simulink model "HighClearancePlant"  (R2016b)
settings: Solver=FixedStepAuto  StartTime=0.0  StopTime=runTime  FixedStep=step_time  MaxStep=0.05  RelTol=1e-3
PreLoadFcn:
  | %load('PlantConfig.mat');
  | run 'PlantParams.m';
values from neighbouring files (symbols this model uses):
  coilMaxI = 0.9*amp2mAmp*Vs/coilR    (= 1800)    [PlantParams.m]
  coilMinI = 0.2*amp2mAmp*Vs/coilR    (= 400)    [PlantParams.m]
  maxFlowRate = maxFlowRate*1    (= 16)    [PlantParams.m]
  reducer_ex = 0.01    [PlantParams.m]
  reducer_rt = 0.01    [PlantParams.m]
  strokeLegnth = 500    [PlantParams.m]
  Vs = 12    [PlantParams.m]
undefined symbols (not defined in the file or in its folder): DiscIntNeverNeededParam, IOD_OK, positionSensor_tblData, positionSensorFL_BrkPnts, positionSensorFR_BrkPnts, positionSensorRL_BrkPnts, positionSensorRR_BrkPnts, trackWidthMin, twoWheelSteer
undefined symbols (not defined in the file): dampeningFL, dampeningFR, extendRateFL, extendRateFR, retractRateFL, retractRateFR
libraries: HighClearance_library x14, PlantLibrary x14, simulink x4
settings Model: Creator=lemaya  LastModifiedBy=lemaya
settings OptimizationCC: DefaultUnderspecifiedDataType=single
settings DebuggingCC: FrameProcessingCompatibilityMsg=warning

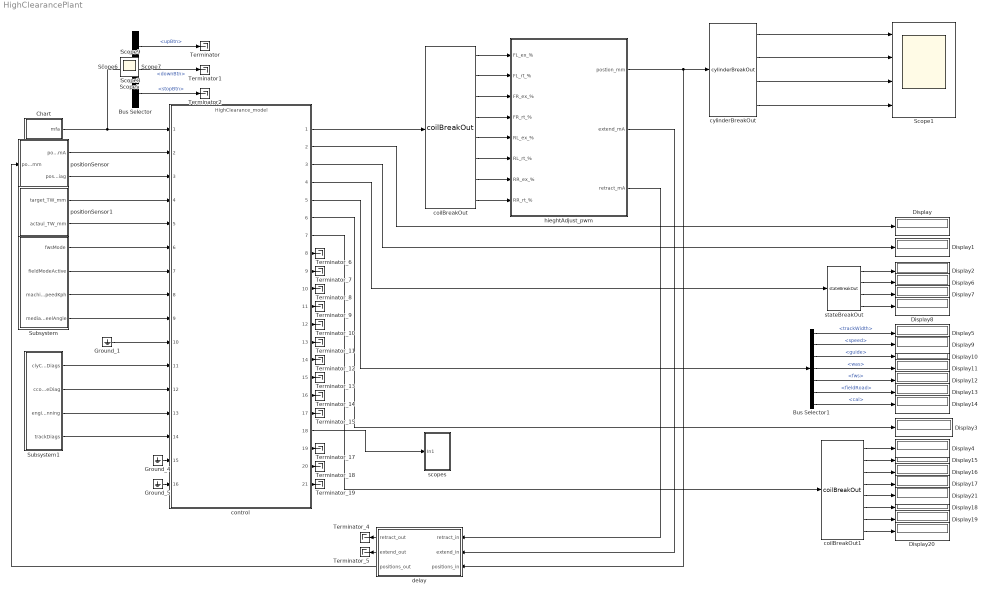
== system HighClearancePlant ==
  Bus Selector : BusSelector  OutputSignals=upBtn,downBtn,stopBtn
  Bus Selector1 : BusSelector  OutputSignals=trackWidth,speed,guide,was,fws,fieldRoad,cal
  Chart : Stateflow chart  TreatAsAtomicUnit=on
  Display{,1..21} (22 alike) : Display
      Display3 settings: Format=hex (Stored Integer)
  Ground_1 : Ground
  Ground_4 : Ground
  Ground_5 : Ground
  Scope1 : Scope  NumInputPorts=4
  Subsystem : Subsystem
  Subsystem1 : Subsystem
  Terminator : Terminator
  Terminator1 : Terminator
  Terminator2 : Terminator
  Terminator_{4..15,17..19} (15 alike) : Terminator
  coilBreakOut : HighClearance_library/coilBreakOut
  coilBreakOut1 : HighClearance_library/coilBreakOut
  control : ModelReference  ModelNameDialog=HighClearance_model.slx  SimulationMode=Normal  ModelReferenceVersion=1.415
  cylinderBreakOut : HighClearance_library/cylinderBreakOut
  delay : Subsystem
  hieghtAdjust_pwm : Subsystem  AncestorBlock=PlantLibrary/hieghtAdjust_pwm
  positionSensor : Subsystem
  positionSensor1 : Subsystem
  scopes : Subsystem
  stateBreakOut : HighClearance_library/stateBreakOut
  Scope{,2..9} (9 alike) : Scope
  wires:
  hieghtAdjust_pwm/2(extend_mA) -> delay/2(extend_in)
  hieghtAdjust_pwm/3(retract_mA) -> delay/1(retract_in)
  hieghtAdjust_pwm/1(postion_mm) -> delay/3(positions_in), cylinderBreakOut/1
  control/1 -> coilBreakOut/1
  positionSensor/1(positions_mA) -> control/2
  delay/3(positions_out) -> positionSensor/1(positons_mm)
  Chart/1(mfa) -> Bus Selector/1, control/1
  coilBreakOut/2 -> hieghtAdjust_pwm/2(FL_rt_%)
  coilBreakOut/3 -> hieghtAdjust_pwm/3(FR_ex_%)
  coilBreakOut/4 -> hieghtAdjust_pwm/4(FR_rt_%)
  coilBreakOut/5 -> hieghtAdjust_pwm/5(RL_ex_%)
  coilBreakOut/6 -> hieghtAdjust_pwm/6(RL_rt_%)
  coilBreakOut/7 -> hieghtAdjust_pwm/7(RR_ex_%)
  coilBreakOut/8 -> hieghtAdjust_pwm/8(RR_rt_%)
  coilBreakOut/1 -> hieghtAdjust_pwm/1(FL_ex_%)
  positionSensor/2(positions_diag) -> control/3
  positionSensor1/1(target_TW_mm) -> control/4
  positionSensor1/2(actaul_TW_mm) -> control/5
  Subsystem/1(fwsMode) -> control/6
  Subsystem/2(fieldModeActive) -> control/7
  Subsystem/3(machineSpeedKph) -> control/8
  Subsystem/4(medianWheelAngle) -> control/9
  Subsystem1/1(clyCoilDiags) -> control/11
  Subsystem1/2(ccoEnableDiag) -> control/12
  control/2 -> Display/1
  control/3 -> Display1/1
  control/4 -> stateBreakOut/1
  control/6 -> Display3/1
  control/7 -> coilBreakOut1/1
  control/5 -> Bus Selector1/1
  Bus Selector/1 -> Terminator/1  "<upBtn>"
  Bus Selector/2 -> Terminator1/1  "<downBtn>"
  Bus Selector/3 -> Terminator2/1  "<stopBtn>"
  Ground_1/1 -> control/10
  delay/1(retract_out) -> Terminator_4/1
  delay/2(extend_out) -> Terminator_5/1
  stateBreakOut/1 -> Display2/1
  stateBreakOut/2 -> Display6/1
  stateBreakOut/3 -> Display7/1
  stateBreakOut/4 -> Display8/1
  Bus Selector1/1 -> Display5/1  "<trackWidth>"
  Bus Selector1/2 -> Display9/1  "<speed>"
  Bus Selector1/3 -> Display10/1  "<guide>"
  Bus Selector1/4 -> Display11/1  "<was>"
  Bus Selector1/5 -> Display12/1  "<fws>"
  Bus Selector1/6 -> Display13/1  "<fieldRoad>"
  Bus Selector1/7 -> Display14/1  "<cal>"
  coilBreakOut1/1 -> Display4/1
  coilBreakOut1/2 -> Display15/1
  coilBreakOut1/3 -> Display16/1
  coilBreakOut1/4 -> Display17/1
  coilBreakOut1/8 -> Display20/1
  coilBreakOut1/7 -> Display19/1
  coilBreakOut1/6 -> Display18/1
  coilBreakOut1/5 -> Display21/1
  cylinderBreakOut/3 -> Scope1/3
  cylinderBreakOut/4 -> Scope1/4
  cylinderBreakOut/2 -> Scope1/2
  cylinderBreakOut/1 -> Scope1/1
  Ground_4/1 -> control/15
  Ground_5/1 -> control/16
  control/8 -> Terminator_6/1
  control/9 -> Terminator_7/1
  control/10 -> Terminator_8/1
  control/11 -> Terminator_9/1
  control/12 -> Terminator_10/1
  control/13 -> Terminator_11/1
  control/14 -> Terminator_12/1
  control/15 -> Terminator_13/1
  control/16 -> Terminator_14/1
  control/17 -> Terminator_15/1
  control/19 -> Terminator_17/1
  control/20 -> Terminator_18/1
  control/21 -> Terminator_19/1
  Subsystem1/3(engineRunning) -> control/13
  Subsystem1/4(trackDiags) -> control/14
  control/18 -> scopes/1(In1)

== system HighClearancePlant/Subsystem ==
  Constant : Constant  Value=twoWheelSteer
  Constant1 : Constant  OutDataTypeStr=Inherit: Inherit via back propagation
  Constant2 : Constant  Value=5  OutDataTypeStr=Inherit: Inherit via back propagation
  Constant3 : Constant  Value=0  OutDataTypeStr=Inherit: Inherit via back propagation
  fwsMode : Outport
  fieldModeActive : Outport  Port=2
  machineSpeedKph : Outport  Port=3
  medianWheelAngle : Outport  Port=4
  wires:
  Constant/1 -> fwsMode/1
  Constant1/1 -> fieldModeActive/1
  Constant2/1 -> machineSpeedKph/1
  Constant3/1 -> medianWheelAngle/1

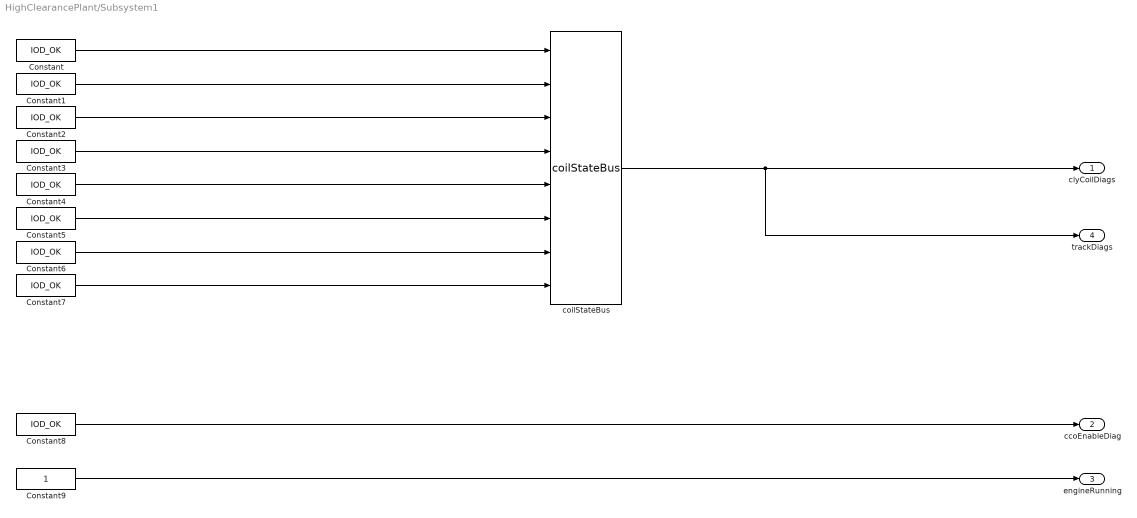
== system HighClearancePlant/Subsystem1 ==
  Constant{,1..8} (9 alike) : Constant  Value=IOD_OK
  Constant9 : Constant  OutDataTypeStr=boolean
  coilStateBus : HighClearance_library/coilStateBus
  clyCoilDiags : Outport
  ccoEnableDiag : Outport  Port=2
  engineRunning : Outport  Port=3
  trackDiags : Outport  Port=4
  wires:
  Constant/1 -> coilStateBus/1
  Constant1/1 -> coilStateBus/2
  Constant2/1 -> coilStateBus/3
  Constant3/1 -> coilStateBus/4
  Constant4/1 -> coilStateBus/5
  Constant5/1 -> coilStateBus/6
  Constant6/1 -> coilStateBus/7
  Constant7/1 -> coilStateBus/8
  coilStateBus/1 -> trackDiags/1, clyCoilDiags/1
  Constant8/1 -> ccoEnableDiag/1
  Constant9/1 -> engineRunning/1

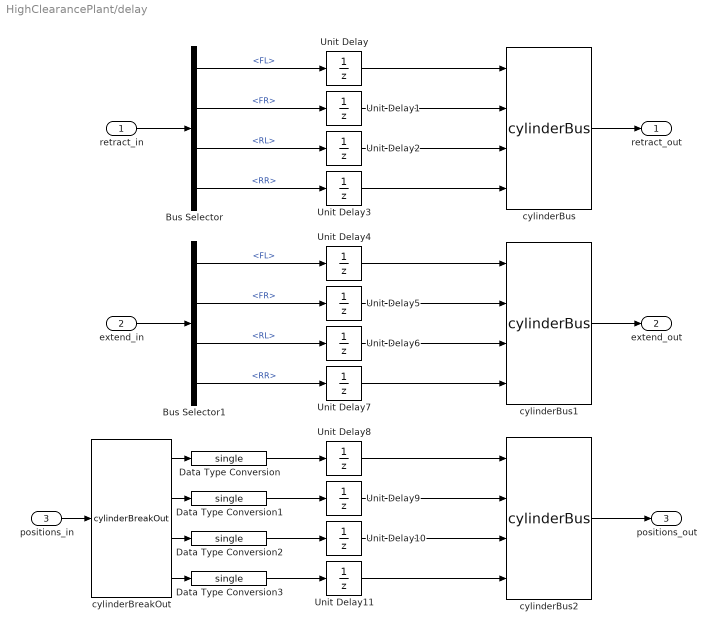
== system HighClearancePlant/delay ==
  retract_in : Inport
  extend_in : Inport  Port=2
  positions_in : Inport  Port=3
  Bus Selector : BusSelector  OutputSignals=FL,FR,RL,RR
  Bus Selector1 : BusSelector  OutputSignals=FL,FR,RL,RR
  Data Type Conversion{,1..3} (4 alike) : DataTypeConversion  OutDataTypeStr=single
  Unit Delay{,1..11} (12 alike) : UnitDelay  SampleTime=-1
  cylinderBreakOut : HighClearance_library/cylinderBreakOut
  cylinderBus : HighClearance_library/cylinderBus
  cylinderBus1 : HighClearance_library/cylinderBus
  cylinderBus2 : HighClearance_library/cylinderBus
  retract_out : Outport
  extend_out : Outport  Port=2
  positions_out : Outport  Port=3
  wires:
  cylinderBus/1 -> retract_out/1
  cylinderBus1/1 -> extend_out/1
  cylinderBus2/1 -> positions_out/1
  retract_in/1 -> Bus Selector/1
  extend_in/1 -> Bus Selector1/1
  Bus Selector1/4 -> Unit Delay7/1  "<RR>"
  Bus Selector1/2 -> Unit Delay5/1  "<FR>"
  Bus Selector1/1 -> Unit Delay4/1  "<FL>"
  Bus Selector1/3 -> Unit Delay6/1  "<RL>"
  Bus Selector/4 -> Unit Delay3/1  "<RR>"
  Bus Selector/1 -> Unit Delay/1  "<FL>"
  Bus Selector/3 -> Unit Delay2/1  "<RL>"
  Bus Selector/2 -> Unit Delay1/1  "<FR>"
  Unit Delay/1 -> cylinderBus/1
  Unit Delay1/1 -> cylinderBus/2
  Unit Delay2/1 -> cylinderBus/3
  Unit Delay3/1 -> cylinderBus/4
  Unit Delay4/1 -> cylinderBus1/1
  Unit Delay7/1 -> cylinderBus1/4
  Unit Delay6/1 -> cylinderBus1/3
  Unit Delay5/1 -> cylinderBus1/2
  Unit Delay8/1 -> cylinderBus2/1
  Unit Delay9/1 -> cylinderBus2/2
  Unit Delay10/1 -> cylinderBus2/3
  Unit Delay11/1 -> cylinderBus2/4
  Data Type Conversion/1 -> Unit Delay8/1
  Data Type Conversion1/1 -> Unit Delay9/1
  Data Type Conversion2/1 -> Unit Delay10/1
  Data Type Conversion3/1 -> Unit Delay11/1
  positions_in/1 -> cylinderBreakOut/1
  cylinderBreakOut/1 -> Data Type Conversion/1
  cylinderBreakOut/2 -> Data Type Conversion1/1
  cylinderBreakOut/3 -> Data Type Conversion2/1
  cylinderBreakOut/4 -> Data Type Conversion3/1

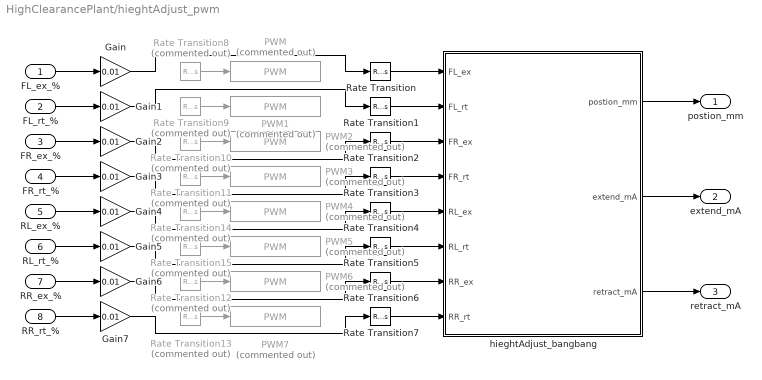
== system HighClearancePlant/hieghtAdjust_pwm ==
  FL_ex_% : Inport
  FL_rt_% : Inport  Port=2
  FR_ex_% : Inport  Port=3
  FR_rt_% : Inport  Port=4
  RL_ex_% : Inport  Port=5
  RL_rt_% : Inport  Port=6
  RR_ex_% : Inport  Port=7
  RR_rt_% : Inport  Port=8
  Gain{,1..7} (8 alike) : Gain  Gain=0.01
  PWM{,1..7} (8 alike) : PlantLibrary/PWM  Commented=on
  Rate Transition{,1..7} (8 alike) : RateTransition
  Rate Transition{8..15} (8 alike) : RateTransition  Commented=on  OutPortSampleTime=0.0001
  hieghtAdjust_bangbang : Subsystem  AncestorBlock=PlantLibrary/hieghtAdjust_bangbang
  postion_mm : Outport
  extend_mA : Outport  Port=2
  retract_mA : Outport  Port=3
  wires:
  Rate Transition7/1 -> hieghtAdjust_bangbang/8(RR_rt)
  Rate Transition6/1 -> hieghtAdjust_bangbang/7(RR_ex)
  Rate Transition5/1 -> hieghtAdjust_bangbang/6(RL_rt)
  Rate Transition4/1 -> hieghtAdjust_bangbang/5(RL_ex)
  Rate Transition3/1 -> hieghtAdjust_bangbang/4(FR_rt)
  Rate Transition2/1 -> hieghtAdjust_bangbang/3(FR_ex)
  Rate Transition1/1 -> hieghtAdjust_bangbang/2(FL_rt)
  Rate Transition/1 -> hieghtAdjust_bangbang/1(FL_ex)
  hieghtAdjust_bangbang/2(extend_mA) -> extend_mA/1
  hieghtAdjust_bangbang/3(retract_mA) -> retract_mA/1
  hieghtAdjust_bangbang/1(postion_mm) -> postion_mm/1
  Rate Transition8/1 -> PWM/1
  Rate Transition9/1 -> PWM1/1
  Rate Transition10/1 -> PWM2/1
  Rate Transition11/1 -> PWM3/1
  Rate Transition14/1 -> PWM4/1
  Rate Transition15/1 -> PWM5/1
  Rate Transition12/1 -> PWM6/1
  Rate Transition13/1 -> PWM7/1
  FL_ex_%/1 -> Gain/1
  FL_rt_%/1 -> Gain1/1
  Gain1/1 -> Rate Transition1/1
  Gain/1 -> Rate Transition/1
  FR_ex_%/1 -> Gain2/1
  Gain2/1 -> Rate Transition2/1
  FR_rt_%/1 -> Gain3/1
  Gain3/1 -> Rate Transition3/1
  RL_ex_%/1 -> Gain4/1
  Gain4/1 -> Rate Transition4/1
  RL_rt_%/1 -> Gain5/1
  Gain5/1 -> Rate Transition5/1
  RR_ex_%/1 -> Gain6/1
  Gain6/1 -> Rate Transition6/1
  RR_rt_%/1 -> Gain7/1
  Gain7/1 -> Rate Transition7/1

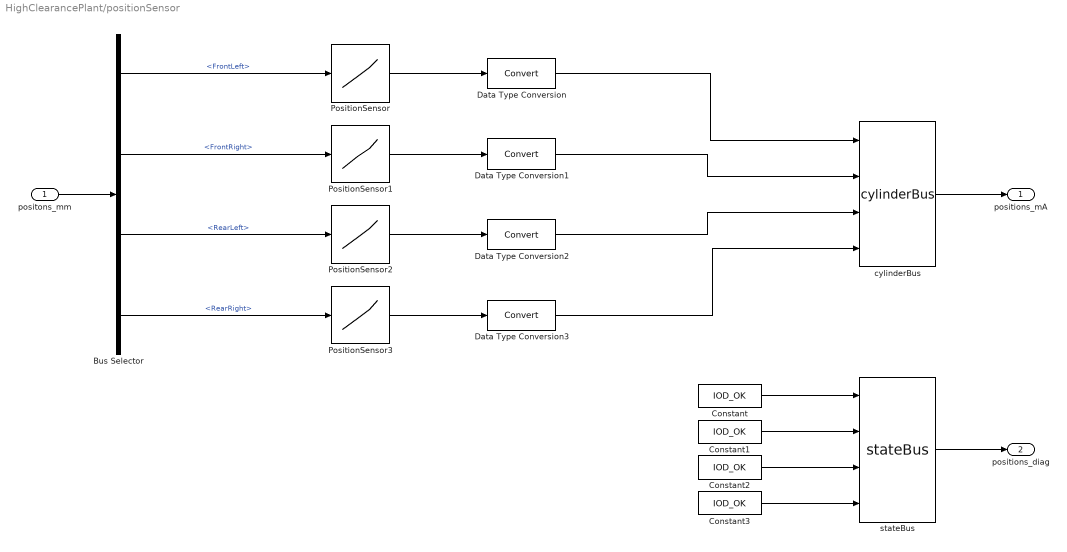
== system HighClearancePlant/positionSensor ==
  positons_mm : Inport
  Bus Selector : BusSelector  OutputSignals=FrontLeft,FrontRight,RearLeft,RearRight
  Constant{,1..3} (4 alike) : Constant  Value=IOD_OK
  Data Type Conversion{,1..3} (4 alike) : DataTypeConversion
  PositionSensor : Lookup_n-D  NumberOfTableDimensions=1  BreakpointsForDimension1=positionSensor_tblData  Table=positionSensorFL_BrkPnts  ExtrapMethod=Clip  UseLastTableValue=on  InternalRulePriority=Speed  RndMeth=Simplest  InputSameDT=on
  PositionSensor1 : Lookup_n-D  NumberOfTableDimensions=1  BreakpointsForDimension1=positionSensor_tblData  Table=positionSensorFR_BrkPnts  ExtrapMethod=Clip  UseLastTableValue=on  InternalRulePriority=Speed  RndMeth=Simplest  InputSameDT=on
  PositionSensor2 : Lookup_n-D  NumberOfTableDimensions=1  BreakpointsForDimension1=positionSensor_tblData  Table=positionSensorRL_BrkPnts  ExtrapMethod=Clip  UseLastTableValue=on  InternalRulePriority=Speed  RndMeth=Simplest  InputSameDT=on
  PositionSensor3 : Lookup_n-D  NumberOfTableDimensions=1  BreakpointsForDimension1=positionSensor_tblData  Table=positionSensorRR_BrkPnts  ExtrapMethod=Clip  UseLastTableValue=on  InternalRulePriority=Speed  RndMeth=Simplest  InputSameDT=on
  cylinderBus : HighClearance_library/cylinderBus
  stateBus : HighClearance_library/stateBus
  positions_mA : Outport  OutDataTypeStr=Bus: CylinderBus
  positions_diag : Outport  Port=2  OutDataTypeStr=Bus: StateBus
  wires:
  positons_mm/1 -> Bus Selector/1
  Bus Selector/1 -> PositionSensor/1  "<FrontLeft>"
  Bus Selector/2 -> PositionSensor1/1  "<FrontRight>"
  Bus Selector/3 -> PositionSensor2/1  "<RearLeft>"
  Bus Selector/4 -> PositionSensor3/1  "<RearRight>"
  PositionSensor/1 -> Data Type Conversion/1
  PositionSensor1/1 -> Data Type Conversion1/1
  PositionSensor2/1 -> Data Type Conversion2/1
  PositionSensor3/1 -> Data Type Conversion3/1
  Data Type Conversion/1 -> cylinderBus/1
  Data Type Conversion1/1 -> cylinderBus/2
  Data Type Conversion2/1 -> cylinderBus/3
  Data Type Conversion3/1 -> cylinderBus/4
  cylinderBus/1 -> positions_mA/1
  stateBus/1 -> positions_diag/1
  Constant/1 -> stateBus/1
  Constant1/1 -> stateBus/2
  Constant2/1 -> stateBus/3
  Constant3/1 -> stateBus/4

== system HighClearancePlant/positionSensor1 ==
  Constant : Constant  Value=trackWidthMin  OutDataTypeStr=Inherit: Inherit via back propagation
  cylinderBus : HighClearance_library/cylinderBus
  cylinderBus1 : HighClearance_library/cylinderBus
  target_TW_mm : Outport  OutDataTypeStr=Bus: CylinderBus
  actaul_TW_mm : Outport  Port=2  OutDataTypeStr=Bus: CylinderBus
  wires:
  cylinderBus1/1 -> actaul_TW_mm/1
  cylinderBus/1 -> target_TW_mm/1
  Constant/1 -> cylinderBus1/4, cylinderBus1/3, cylinderBus1/2, cylinderBus1/1, cylinderBus/4, cylinderBus/3, cylinderBus/2, cylinderBus/1

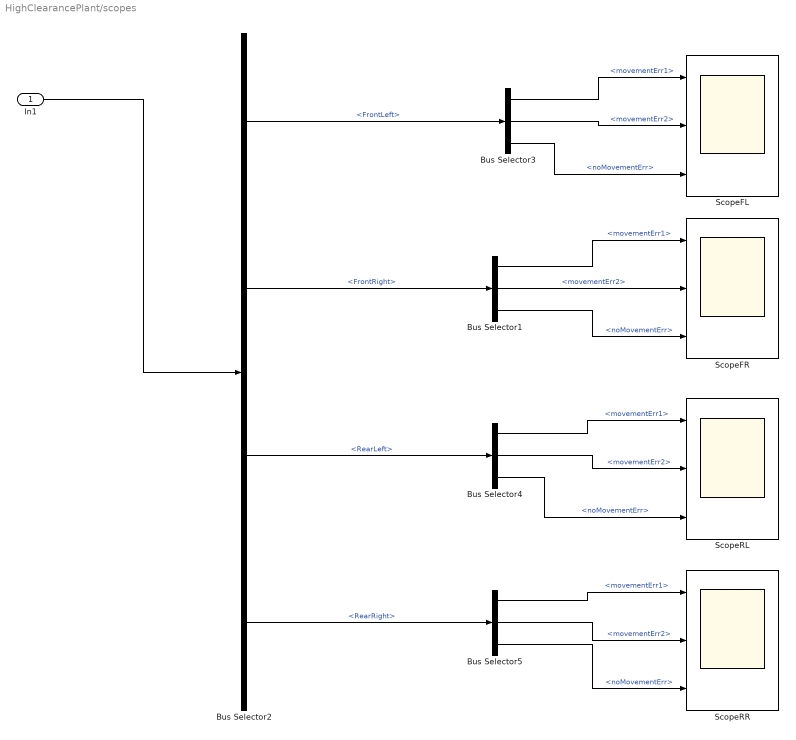
== system HighClearancePlant/scopes ==
  In1 : Inport
  Bus Selector{1,3..5} (4 alike) : BusSelector  OutputSignals=movementErr1,movementErr2,noMovementErr
  Bus Selector2 : BusSelector  OutputSignals=FrontLeft,FrontRight,RearLeft,RearRight
  ScopeFL : Scope  NumInputPorts=3
  ScopeFR : Scope  NumInputPorts=3
  ScopeRL : Scope  NumInputPorts=3
  ScopeRR : Scope  NumInputPorts=3
  wires:
  In1/1 -> Bus Selector2/1
  Bus Selector2/1 -> Bus Selector3/1  "<FrontLeft>"
  Bus Selector2/2 -> Bus Selector1/1  "<FrontRight>"
  Bus Selector2/3 -> Bus Selector4/1  "<RearLeft>"
  Bus Selector2/4 -> Bus Selector5/1  "<RearRight>"
  Bus Selector3/2 -> ScopeFL/2  "<movementErr2>"
  Bus Selector3/1 -> ScopeFL/1  "<movementErr1>"
  Bus Selector3/3 -> ScopeFL/3  "<noMovementErr>"
  Bus Selector1/2 -> ScopeFR/2  "<movementErr2>"
  Bus Selector1/3 -> ScopeFR/3  "<noMovementErr>"
  Bus Selector1/1 -> ScopeFR/1  "<movementErr1>"
  Bus Selector4/2 -> ScopeRL/2  "<movementErr2>"
  Bus Selector4/1 -> ScopeRL/1  "<movementErr1>"
  Bus Selector4/3 -> ScopeRL/3  "<noMovementErr>"
  Bus Selector5/1 -> ScopeRR/1  "<movementErr1>"
  Bus Selector5/2 -> ScopeRR/2  "<movementErr2>"
  Bus Selector5/3 -> ScopeRR/3  "<noMovementErr>"

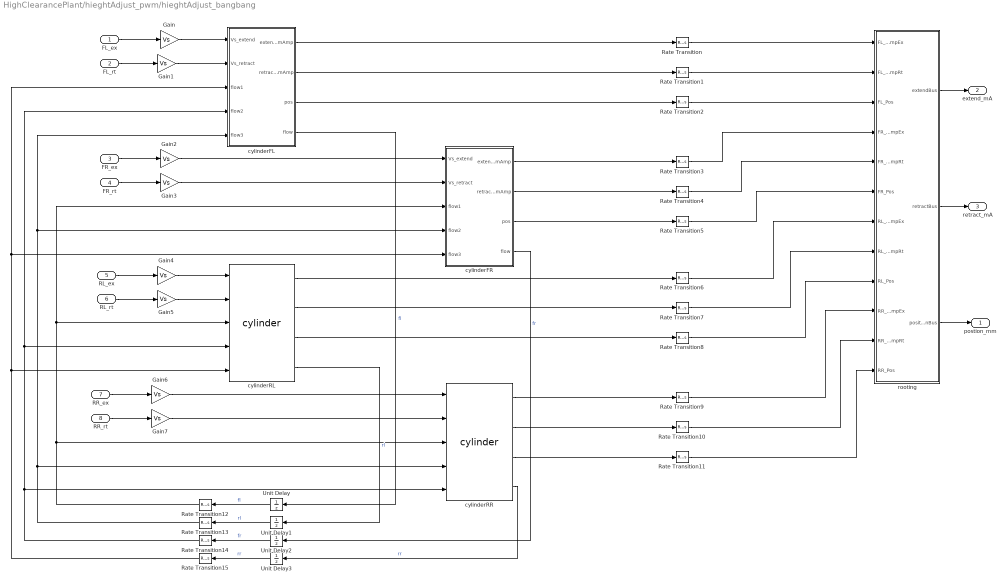
== system HighClearancePlant/hieghtAdjust_pwm/hieghtAdjust_bangbang ==
  FL_ex : Inport
  FL_rt : Inport  Port=2
  FR_ex : Inport  Port=3
  FR_rt : Inport  Port=4
  RL_ex : Inport  Port=5
  RL_rt : Inport  Port=6
  RR_ex : Inport  Port=7
  RR_rt : Inport  Port=8
  Gain{,1..7} (8 alike) : Gain  Gain=Vs
  Rate Transition{,1..11,13..15} (15 alike) : RateTransition  OutPortSampleTime=step_time
  Rate Transition12 : RateTransition
  Unit Delay{,1..3} (4 alike) : UnitDelay  SampleTime=-1
  cylinderFL : Subsystem  AncestorBlock=PlantLibrary/cylinder  mask{dampening=dampeningFL, extendRate=extendRateFL, retractRate=retractRateFL}
      mask prompts: dampening "Dampening coefficient:"; extendRate "Extend Rate [mm/sec]:"; retractRate "Retract Rate [mm/sec]:"
  cylinderFR : Subsystem  AncestorBlock=PlantLibrary/cylinder  mask{dampening=dampeningFR, extendRate=extendRateFR, retractRate=retractRateFR}
      mask prompts: dampening "Dampening coefficient:"; extendRate "Extend Rate [mm/sec]:"; retractRate "Retract Rate [mm/sec]:"
  cylinderRL : PlantLibrary/cylinder  dampening=dampeningRL  extendRate=extendRateRL  retractRate=retractRateRL
  cylinderRR : PlantLibrary/cylinder  dampening=dampeningRR  extendRate=extendRateRR  retractRate=retractRateRR
  rooting : Subsystem
  postion_mm : Outport
  extend_mA : Outport  Port=2
  retract_mA : Outport  Port=3
  wires:
  cylinderRR/2 -> Rate Transition10/1
  cylinderRR/1 -> Rate Transition9/1
  cylinderRL/2 -> Rate Transition7/1
  cylinderRL/1 -> Rate Transition6/1
  cylinderFR/2(retract_mAmp) -> Rate Transition4/1
  cylinderFR/1(extend_mAmp) -> Rate Transition3/1
  cylinderFL/2(retract_mAmp) -> Rate Transition1/1
  cylinderFL/1(extend_mAmp) -> Rate Transition/1
  rooting/3(positionBus) -> postion_mm/1
  rooting/2(retractBus) -> retract_mA/1
  rooting/1(extendBus) -> extend_mA/1
  FL_rt/1 -> Gain1/1
  RR_rt/1 -> Gain7/1
  RL_ex/1 -> Gain4/1
  FL_ex/1 -> Gain/1
  FR_ex/1 -> Gain2/1
  FR_rt/1 -> Gain3/1
  RR_ex/1 -> Gain6/1
  RL_rt/1 -> Gain5/1
  Gain/1 -> cylinderFL/1(Vs_extend)
  Gain1/1 -> cylinderFL/2(Vs_retract)
  Gain4/1 -> cylinderRL/1
  Gain5/1 -> cylinderRL/2
  Gain6/1 -> cylinderRR/1
  Gain7/1 -> cylinderRR/2
  Rate Transition/1 -> rooting/1(FL_mAmpEx)
  Rate Transition1/1 -> rooting/2(FL_mAmpRt)
  Rate Transition2/1 -> rooting/3(FL_Pos)
  Rate Transition3/1 -> rooting/4(FR_mAmpEx)
  Rate Transition4/1 -> rooting/5(FR_mAmpRt)
  Rate Transition5/1 -> rooting/6(FR_Pos)
  Rate Transition6/1 -> rooting/7(RL_mAmpEx)
  Rate Transition7/1 -> rooting/8(RL_mAmpRt)
  Rate Transition8/1 -> rooting/9(RL_Pos)
  Rate Transition9/1 -> rooting/10(RR_mAmpEx)
  Rate Transition10/1 -> rooting/11(RR_mAmpRt)
  Rate Transition11/1 -> rooting/12(RR_Pos)
  cylinderFL/3(pos) -> Rate Transition2/1
  cylinderRL/3 -> Rate Transition8/1
  cylinderFR/3(pos) -> Rate Transition5/1
  cylinderRR/3 -> Rate Transition11/1
  Gain3/1 -> cylinderFR/2(Vs_retract)
  Gain2/1 -> cylinderFR/1(Vs_extend)
  cylinderRL/4 -> Unit Delay1/1  "rl"
  cylinderFR/4(flow) -> Unit Delay2/1  "fr"
  cylinderRR/4 -> Unit Delay3/1  "rr"
  cylinderFL/4(flow) -> Unit Delay/1  "fl"
  Unit Delay/1 -> Rate Transition12/1  "fl"
  Unit Delay3/1 -> Rate Transition15/1  "rr"
  Unit Delay2/1 -> Rate Transition14/1  "fr"
  Unit Delay1/1 -> Rate Transition13/1  "rl"
  Rate Transition12/1 -> cylinderFR/3(flow1), cylinderRL/3, cylinderRR/3
  Rate Transition13/1 -> cylinderFL/5(flow3), cylinderFR/4(flow2), cylinderRR/4
  Rate Transition14/1 -> cylinderFL/4(flow2), cylinderRL/4, cylinderRR/5
  Rate Transition15/1 -> cylinderRL/5, cylinderFL/3(flow1), cylinderFR/5(flow3)

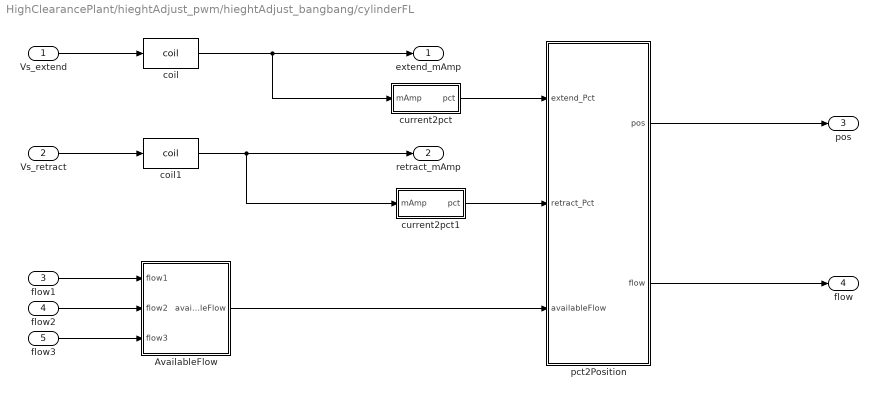
== system HighClearancePlant/hieghtAdjust_pwm/hieghtAdjust_bangbang/cylinderFL ==
  Vs_extend : Inport
  Vs_retract : Inport  Port=2
  flow1 : Inport  Port=3
  flow2 : Inport  Port=4
  flow3 : Inport  Port=5
  AvailableFlow : Subsystem
  coil : PlantLibrary/coil
  coil1 : PlantLibrary/coil
  current2pct : Subsystem
  current2pct1 : Subsystem
  pct2Position : Subsystem
  extend_mAmp : Outport
  retract_mAmp : Outport  Port=2
  pos : Outport  Port=3
  flow : Outport  Port=4
  wires:
  Vs_extend/1 -> coil/1
  Vs_retract/1 -> coil1/1
  coil/1 -> current2pct/1(mAmp), extend_mAmp/1
  coil1/1 -> current2pct1/1(mAmp), retract_mAmp/1
  current2pct/1(pct) -> pct2Position/1(extend_Pct)
  current2pct1/1(pct) -> pct2Position/2(retract_Pct)
  pct2Position/1(pos) -> pos/1
  pct2Position/2(flow) -> flow/1
  flow1/1 -> AvailableFlow/1(flow1)
  flow2/1 -> AvailableFlow/2(flow2)
  flow3/1 -> AvailableFlow/3(flow3)
  AvailableFlow/1(availableFlow) -> pct2Position/3(availableFlow)

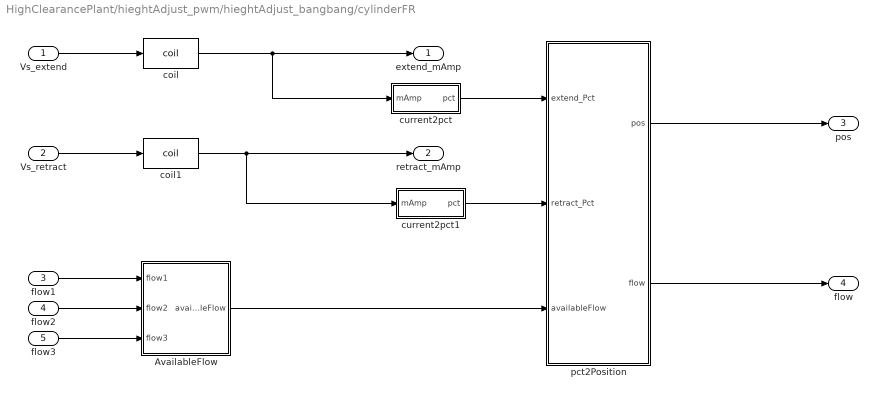
== system HighClearancePlant/hieghtAdjust_pwm/hieghtAdjust_bangbang/cylinderFR ==
  Vs_extend : Inport
  Vs_retract : Inport  Port=2
  flow1 : Inport  Port=3
  flow2 : Inport  Port=4
  flow3 : Inport  Port=5
  AvailableFlow : Subsystem
  coil : PlantLibrary/coil
  coil1 : PlantLibrary/coil
  current2pct : Subsystem
  current2pct1 : Subsystem
  pct2Position : Subsystem
  extend_mAmp : Outport
  retract_mAmp : Outport  Port=2
  pos : Outport  Port=3
  flow : Outport  Port=4
  wires:
  Vs_extend/1 -> coil/1
  Vs_retract/1 -> coil1/1
  coil/1 -> current2pct/1(mAmp), extend_mAmp/1
  coil1/1 -> current2pct1/1(mAmp), retract_mAmp/1
  current2pct/1(pct) -> pct2Position/1(extend_Pct)
  current2pct1/1(pct) -> pct2Position/2(retract_Pct)
  pct2Position/1(pos) -> pos/1
  pct2Position/2(flow) -> flow/1
  flow1/1 -> AvailableFlow/1(flow1)
  flow2/1 -> AvailableFlow/2(flow2)
  flow3/1 -> AvailableFlow/3(flow3)
  AvailableFlow/1(availableFlow) -> pct2Position/3(availableFlow)

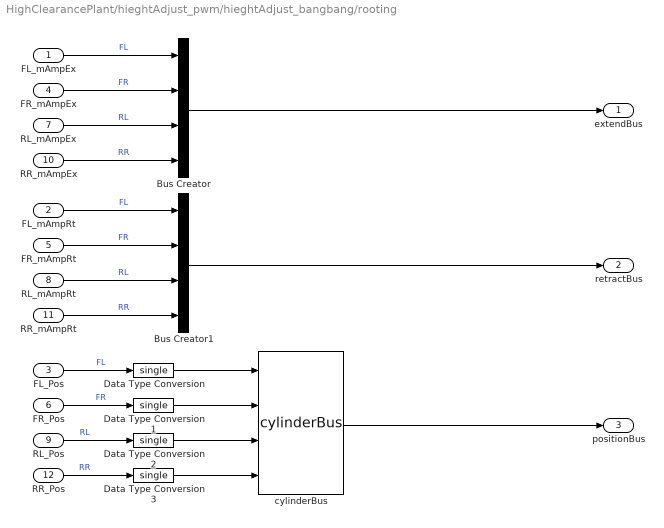
== system HighClearancePlant/hieghtAdjust_pwm/hieghtAdjust_bangbang/rooting ==
  FL_mAmpEx : Inport
  FL_mAmpRt : Inport  Port=2
  FL_Pos : Inport  Port=3
  FR_mAmpEx : Inport  Port=4
  FR_mAmpRt : Inport  Port=5
  FR_Pos : Inport  Port=6
  RL_mAmpEx : Inport  Port=7
  RL_mAmpRt : Inport  Port=8
  RL_Pos : Inport  Port=9
  RR_mAmpEx : Inport  Port=10
  RR_mAmpRt : Inport  Port=11
  RR_Pos : Inport  Port=12
  Bus Creator : BusCreator  Inputs=4
  Bus Creator1 : BusCreator  Inputs=4
  Data Type Conversion{,1..3} (4 alike) : DataTypeConversion  OutDataTypeStr=single
  cylinderBus : HighClearance_library/cylinderBus
  extendBus : Outport
  retractBus : Outport  Port=2
  positionBus : Outport  Port=3
  wires:
  Bus Creator1/1 -> retractBus/1
  Bus Creator/1 -> extendBus/1
  RR_mAmpRt/1 -> Bus Creator1/4  "RR"
  RL_mAmpRt/1 -> Bus Creator1/3  "RL"
  FR_mAmpRt/1 -> Bus Creator1/2  "FR"
  FL_mAmpRt/1 -> Bus Creator1/1  "FL"
  RR_mAmpEx/1 -> Bus Creator/4  "RR"
  RL_mAmpEx/1 -> Bus Creator/3  "RL"
  FR_mAmpEx/1 -> Bus Creator/2  "FR"
  FL_mAmpEx/1 -> Bus Creator/1  "FL"
  cylinderBus/1 -> positionBus/1
  Data Type Conversion/1 -> cylinderBus/1
  Data Type Conversion1/1 -> cylinderBus/2
  Data Type Conversion2/1 -> cylinderBus/3
  Data Type Conversion3/1 -> cylinderBus/4
  FL_Pos/1 -> Data Type Conversion/1  "FL"
  FR_Pos/1 -> Data Type Conversion1/1  "FR"
  RL_Pos/1 -> Data Type Conversion2/1  "RL"
  RR_Pos/1 -> Data Type Conversion3/1  "RR"

== system HighClearancePlant/hieghtAdjust_pwm/hieghtAdjust_bangbang/cylinderFL/AvailableFlow ==
  flow1 : Inport
  flow2 : Inport  Port=2
  flow3 : Inport  Port=3
  Constant : Constant  Value=maxFlowRate
  Saturation : Saturate  UpperLimit=0  LowerLimit=-inf
  Subtract : Sum  Inputs=+-
  Sum : Sum  Inputs=+++
  availableFlow : Outport
  wires:
  flow3/1 -> Sum/3
  flow1/1 -> Sum/1
  Constant/1 -> Subtract/1
  flow2/1 -> Sum/2
  Sum/1 -> Subtract/2
  Subtract/1 -> Saturation/1
  Saturation/1 -> availableFlow/1

== system HighClearancePlant/hieghtAdjust_pwm/hieghtAdjust_bangbang/cylinderFL/current2pct ==
  mAmp : Inport
  Divide1 : Product  Inputs=*/
  Gain : Gain  Gain=100
  Relational Operator : RelationalOperator  OutDataTypeStr=boolean  RndMeth=Simplest
  Saturation : Saturate  UpperLimit=100  LowerLimit=0
  Switch : Switch  Criteria=u2 > Threshold
  maxCurrent : Constant  Value=coilMaxI
  minCurrent : Constant  Value=coilMinI
  pct : Outport
  wires:
  maxCurrent/1 -> Divide1/2
  Relational Operator/1 -> Switch/3, Switch/2
  minCurrent/1 -> Relational Operator/2
  Switch/1 -> Divide1/1
  mAmp/1 -> Relational Operator/1, Switch/1
  Divide1/1 -> Gain/1
  Saturation/1 -> pct/1
  Gain/1 -> Saturation/1

== system HighClearancePlant/hieghtAdjust_pwm/hieghtAdjust_bangbang/cylinderFL/current2pct1 ==
  mAmp : Inport
  Divide1 : Product  Inputs=*/
  Gain : Gain  Gain=100
  Relational Operator : RelationalOperator  OutDataTypeStr=boolean  RndMeth=Simplest
  Saturation : Saturate  UpperLimit=100  LowerLimit=0
  Switch : Switch  Criteria=u2 > Threshold
  maxCurrent : Constant  Value=coilMaxI
  minCurrent : Constant  Value=coilMinI
  pct : Outport
  wires:
  Gain/1 -> Saturation/1
  Saturation/1 -> pct/1
  Divide1/1 -> Gain/1
  mAmp/1 -> Switch/1, Relational Operator/1
  Switch/1 -> Divide1/1
  minCurrent/1 -> Relational Operator/2
  Relational Operator/1 -> Switch/2, Switch/3
  maxCurrent/1 -> Divide1/2

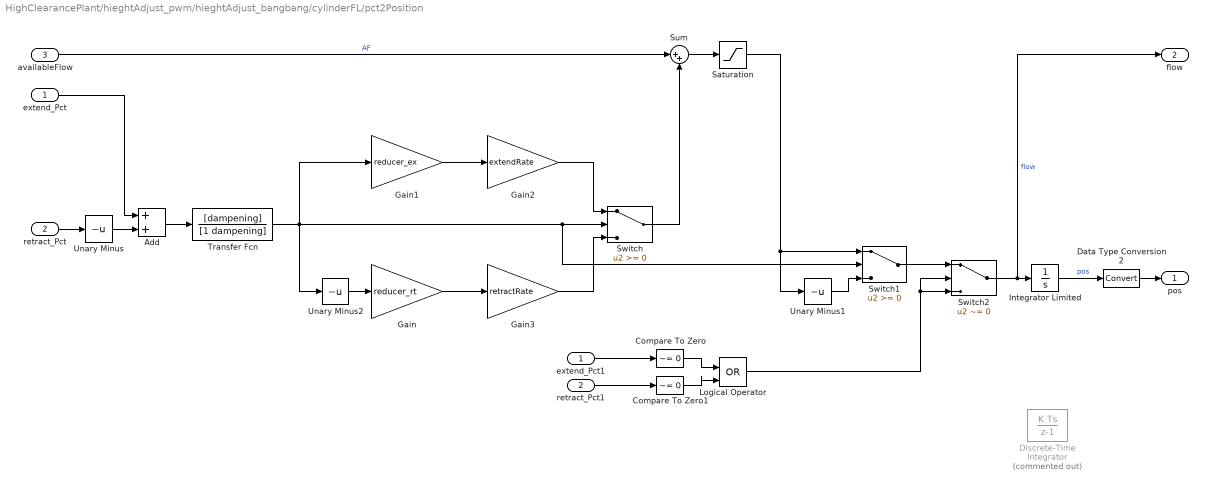
== system HighClearancePlant/hieghtAdjust_pwm/hieghtAdjust_bangbang/cylinderFL/pct2Position ==
  extend_Pct : Inport
  retract_Pct : Inport  Port=2
  availableFlow : Inport  Port=3
  Add : Sum  SaturateOnIntegerOverflow=on
  Compare To Zero : simulink/Logic and Bit Operations/Compare To Zero  relop=~=  OutDataTypeStr=boolean
  Compare To Zero1 : simulink/Logic and Bit Operations/Compare To Zero  relop=~=  OutDataTypeStr=boolean
  Data Type Conversion2 : DataTypeConversion
  Discrete-Time Integrator : DiscreteIntegrator  Commented=on  InitialConditionSetting=State (most efficient)  SampleTime=-1  LimitOutput=on  UpperSaturationLimit=strokeLegnth  LowerSaturationLimit=0  ICPrevOutput=DiscIntNeverNeededParam  ICPrevScaledInput=DiscIntNeverNeededParam
  Gain : Gain  Gain=reducer_rt  OutDataTypeStr=single  SaturateOnIntegerOverflow=on
  Gain1 : Gain  Gain=reducer_ex  OutDataTypeStr=single  SaturateOnIntegerOverflow=on
  Gain2 : Gain  Gain=extendRate  OutDataTypeStr=single  SaturateOnIntegerOverflow=on
  Gain3 : Gain  Gain=retractRate  OutDataTypeStr=single  SaturateOnIntegerOverflow=on
  Integrator Limited : Integrator  LimitOutput=on  UpperSaturationLimit=strokeLegnth  LowerSaturationLimit=0
  Logical Operator : Logic  Operator=OR  IconShape=distinctive  AllPortsSameDT=off  OutDataTypeStr=boolean
  Saturation : Saturate  UpperLimit=inf  LowerLimit=0
  Sum : Sum  Inputs=|++
  Switch : Switch  OutDataTypeStr=Inherit: Inherit via back propagation  SaturateOnIntegerOverflow=on
  Switch1 : Switch  OutDataTypeStr=Inherit: Inherit via back propagation  SaturateOnIntegerOverflow=on
  Switch2 : Switch  Criteria=u2 ~= 0  OutDataTypeStr=Inherit: Inherit via back propagation  SaturateOnIntegerOverflow=on
  Transfer Fcn : TransferFcn  Numerator=[dampening]  Denominator=[1 dampening]
  Unary Minus : UnaryMinus  SaturateOnIntegerOverflow=on
  Unary Minus1 : UnaryMinus  SaturateOnIntegerOverflow=on
  Unary Minus2 : UnaryMinus  SaturateOnIntegerOverflow=on
  extend_Pct1 : InportShadow
  retract_Pct1 : InportShadow  Port=2
  pos : Outport
  flow : Outport  Port=2
  wires:
  Gain/1 -> Gain3/1
  Gain1/1 -> Gain2/1
  Data Type Conversion2/1 -> pos/1
  retract_Pct/1 -> Unary Minus/1
  Unary Minus/1 -> Add/2
  extend_Pct/1 -> Add/1
  Add/1 -> Transfer Fcn/1
  Sum/1 -> Saturation/1
  Gain2/1 -> Switch/1
  Gain3/1 -> Switch/3
  Integrator Limited/1 -> Data Type Conversion2/1  "pos"
  availableFlow/1 -> Sum/1  "AF"
  Switch/1 -> Sum/2
  Unary Minus2/1 -> Gain/1
  Transfer Fcn/1 -> Switch/2, Switch1/2, Unary Minus2/1, Gain1/1
  Switch1/1 -> Switch2/1
  Unary Minus1/1 -> Switch1/3
  Saturation/1 -> Unary Minus1/1, Switch1/1
  extend_Pct1/1 -> Compare To Zero/1
  retract_Pct1/1 -> Compare To Zero1/1
  Compare To Zero/1 -> Logical Operator/1
  Compare To Zero1/1 -> Logical Operator/2
  Logical Operator/1 -> Switch2/3, Switch2/2
  Switch2/1 -> flow/1, Integrator Limited/1  "flow"

== system HighClearancePlant/hieghtAdjust_pwm/hieghtAdjust_bangbang/cylinderFR/AvailableFlow ==
  flow1 : Inport
  flow2 : Inport  Port=2
  flow3 : Inport  Port=3
  Constant : Constant  Value=maxFlowRate
  Saturation : Saturate  UpperLimit=0  LowerLimit=-inf
  Subtract : Sum  Inputs=+-
  Sum : Sum  Inputs=+++
  availableFlow : Outport
  wires:
  flow3/1 -> Sum/3
  flow1/1 -> Sum/1
  Constant/1 -> Subtract/1
  flow2/1 -> Sum/2
  Sum/1 -> Subtract/2
  Subtract/1 -> Saturation/1
  Saturation/1 -> availableFlow/1

== system HighClearancePlant/hieghtAdjust_pwm/hieghtAdjust_bangbang/cylinderFR/current2pct ==
  mAmp : Inport
  Divide1 : Product  Inputs=*/
  Gain : Gain  Gain=100
  Relational Operator : RelationalOperator  OutDataTypeStr=boolean  RndMeth=Simplest
  Saturation : Saturate  UpperLimit=100  LowerLimit=0
  Switch : Switch  Criteria=u2 > Threshold
  maxCurrent : Constant  Value=coilMaxI
  minCurrent : Constant  Value=coilMinI
  pct : Outport
  wires:
  maxCurrent/1 -> Divide1/2
  Relational Operator/1 -> Switch/3, Switch/2
  minCurrent/1 -> Relational Operator/2
  Switch/1 -> Divide1/1
  mAmp/1 -> Relational Operator/1, Switch/1
  Divide1/1 -> Gain/1
  Saturation/1 -> pct/1
  Gain/1 -> Saturation/1

== system HighClearancePlant/hieghtAdjust_pwm/hieghtAdjust_bangbang/cylinderFR/current2pct1 ==
  mAmp : Inport
  Divide1 : Product  Inputs=*/
  Gain : Gain  Gain=100
  Relational Operator : RelationalOperator  OutDataTypeStr=boolean  RndMeth=Simplest
  Saturation : Saturate  UpperLimit=100  LowerLimit=0
  Switch : Switch  Criteria=u2 > Threshold
  maxCurrent : Constant  Value=coilMaxI
  minCurrent : Constant  Value=coilMinI
  pct : Outport
  wires:
  Gain/1 -> Saturation/1
  Saturation/1 -> pct/1
  Divide1/1 -> Gain/1
  mAmp/1 -> Switch/1, Relational Operator/1
  Switch/1 -> Divide1/1
  minCurrent/1 -> Relational Operator/2
  Relational Operator/1 -> Switch/2, Switch/3
  maxCurrent/1 -> Divide1/2

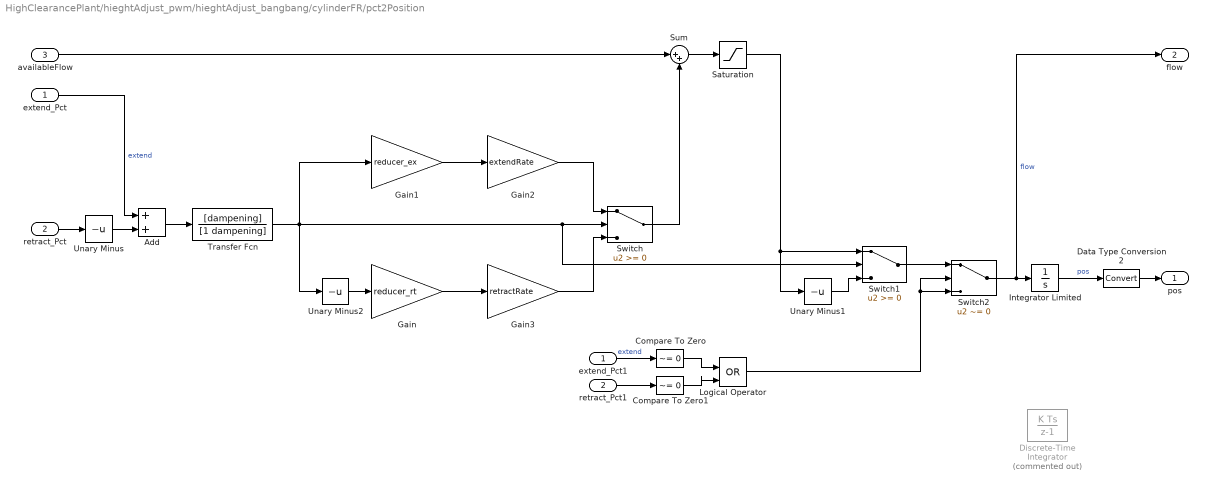
== system HighClearancePlant/hieghtAdjust_pwm/hieghtAdjust_bangbang/cylinderFR/pct2Position ==
  extend_Pct : Inport
  retract_Pct : Inport  Port=2
  availableFlow : Inport  Port=3
  Add : Sum  SaturateOnIntegerOverflow=on
  Compare To Zero : simulink/Logic and Bit Operations/Compare To Zero  relop=~=  OutDataTypeStr=boolean
  Compare To Zero1 : simulink/Logic and Bit Operations/Compare To Zero  relop=~=  OutDataTypeStr=boolean
  Data Type Conversion2 : DataTypeConversion
  Discrete-Time Integrator : DiscreteIntegrator  Commented=on  InitialConditionSetting=State (most efficient)  SampleTime=-1  LimitOutput=on  UpperSaturationLimit=strokeLegnth  LowerSaturationLimit=0  ICPrevOutput=DiscIntNeverNeededParam  ICPrevScaledInput=DiscIntNeverNeededParam
  Gain : Gain  Gain=reducer_rt  OutDataTypeStr=single  SaturateOnIntegerOverflow=on
  Gain1 : Gain  Gain=reducer_ex  OutDataTypeStr=single  SaturateOnIntegerOverflow=on
  Gain2 : Gain  Gain=extendRate  OutDataTypeStr=single  SaturateOnIntegerOverflow=on
  Gain3 : Gain  Gain=retractRate  OutDataTypeStr=single  SaturateOnIntegerOverflow=on
  Integrator Limited : Integrator  LimitOutput=on  UpperSaturationLimit=strokeLegnth  LowerSaturationLimit=0
  Logical Operator : Logic  Operator=OR  IconShape=distinctive  AllPortsSameDT=off  OutDataTypeStr=boolean
  Saturation : Saturate  UpperLimit=inf  LowerLimit=0
  Sum : Sum  Inputs=|++
  Switch : Switch  OutDataTypeStr=Inherit: Inherit via back propagation  SaturateOnIntegerOverflow=on
  Switch1 : Switch  OutDataTypeStr=Inherit: Inherit via back propagation  SaturateOnIntegerOverflow=on
  Switch2 : Switch  Criteria=u2 ~= 0  OutDataTypeStr=Inherit: Inherit via back propagation  SaturateOnIntegerOverflow=on
  Transfer Fcn : TransferFcn  Numerator=[dampening]  Denominator=[1 dampening]
  Unary Minus : UnaryMinus  SaturateOnIntegerOverflow=on
  Unary Minus1 : UnaryMinus  SaturateOnIntegerOverflow=on
  Unary Minus2 : UnaryMinus  SaturateOnIntegerOverflow=on
  extend_Pct1 : InportShadow
  retract_Pct1 : InportShadow  Port=2
  pos : Outport
  flow : Outport  Port=2
  wires:
  Gain/1 -> Gain3/1
  Gain1/1 -> Gain2/1
  Data Type Conversion2/1 -> pos/1
  retract_Pct/1 -> Unary Minus/1
  Unary Minus/1 -> Add/2
  extend_Pct/1 -> Add/1  "extend"
  Add/1 -> Transfer Fcn/1
  Sum/1 -> Saturation/1
  Gain2/1 -> Switch/1
  Gain3/1 -> Switch/3
  Integrator Limited/1 -> Data Type Conversion2/1  "pos"
  availableFlow/1 -> Sum/1
  Switch/1 -> Sum/2
  Unary Minus2/1 -> Gain/1
  Transfer Fcn/1 -> Switch/2, Switch1/2, Unary Minus2/1, Gain1/1
  Switch1/1 -> Switch2/1
  Unary Minus1/1 -> Switch1/3
  Saturation/1 -> Unary Minus1/1, Switch1/1
  extend_Pct1/1 -> Compare To Zero/1  "extend"
  retract_Pct1/1 -> Compare To Zero1/1
  Compare To Zero/1 -> Logical Operator/1
  Compare To Zero1/1 -> Logical Operator/2
  Logical Operator/1 -> Switch2/3, Switch2/2
  Switch2/1 -> flow/1, Integrator Limited/1  "flow"

== stateflow chart HighClearancePlant/Chart ==
  state step
    en: mfa.upBtn = 0;
  state step1
    en: mfa.upBtn = 1;
  state step2
    en: mfa.upBtn = 0;
  (default) -> step
  step1 -> step2 : after(50,msec)
  step -> step1 : after(1,sec)
  data: mfa output Bus: MfaBus
